simulink model "quadplane_control_dev"  (R2023a)
settings: Solver=FixedStepAuto  StartTime=0.0  StopTime=10.0  FixedStep=0.01  RelTol=1e-3
undefined symbols (not defined in the file or in its folder): Aircraft, DiscIntNeverNeededParam, framePeriod_s, frameRate_hz, InitCond
libraries: simulink x8, eeGeneralControl x6, slpidlib x3, fuzblock x1
(part 3 of 3)

== matlab function quadplane_control_dev/LowPass Filter2/LP Filter on throttle outputs/MATLAB Function ==
  data: prev_val input single; raw_val input; filtered_val output; freq_cut input; samp_freq input
function filtered_val = IIR_filt( prev_val,raw_val, freq_cut, samp_freq)
    fc = freq_cut/samp_freq;
    b = 2 - cos(2 * pi * fc) - sqrt((2 - cos(2 * pi * fc))^2 - 1);
    a = 1 - b;
    filtered_val = a * raw_val + b * prev_val;

== matlab function quadplane_control_dev/Hover Inner Loop/INDI inner loop/MATLAB Function ==
  data: B0_mat input; motor_cmds output; x_ref_rate input; Kp_term input; x_rate input
function motor_cmds = indi_inner_control(B0_mat, x_ref_rate, Kp_term, x_rate)

% INDI output change equation
motor_cmds = B0_mat \ (-x_rate + Kp_term + x_ref_rate);

== matlab function quadplane_control_dev/Hover Inner Loop/INDI inner loop/MATLAB Function1 ==
  data: mass input; cg_pos input; thrust_coefs input; B0_mat output; torque_coefs input; motor_pos input; new_inertia_inv input; motor_cmds input
function B0_mat = inversion_matrix(mass, cg_pos, thrust_coefs, torque_coefs, motor_pos, new_inertia_inv, motor_cmds)
% Included all moments modelled for hover flight

% Assumed thrust coefficient and torque coefficients are 2nd order. 
moment_arm = motor_pos - cg_pos';

% 2*a1*omega_i + a2
dummy_term = 2 * thrust_coefs(1) .* motor_cmds' + thrust_coefs(2);

% dummy term with respective y position of motor
row_1_term = - moment_arm(1:4, 2)' .* dummy_term;

% dummy term with respective x position of motor
row_2_term = moment_arm(1:4, 1)' .* dummy_term;

% 2*b1*omega_i + b2
row_3_term = [-1,-1,1,1] .* (2 * torque_coefs(1) .* motor_cmds' + torque_coefs(2));

% (-1/m)(2a1*omega_i+a2)
row_4_term = (-1/mass) * (dummy_term);

% inversion matrix for INDI
B0_mat = new_inertia_inv * [row_1_term; row_2_term; row_3_term; row_4_term];

== matlab function quadplane_control_dev/Frame Conversion ==
  data: ned_vector input; rpy_euler input; body_vector output
function body_vector = ned2body(ned_vector, rpy_euler)

roll = rpy_euler(1);
pitch = rpy_euler(2);
yaw = rpy_euler(3);

% Rotation matrix from NED to Body frame
C_ned2body = [cos(pitch)*cos(yaw), cos(pitch)*sin(yaw), -sin(pitch); ...
    sin(roll)*sin(pitch)*cos(yaw)-cos(roll)*sin(yaw), ...
    sin(roll)*sin(pitch)*sin(yaw)+cos(roll)*cos(yaw), sin(roll)*cos(pitch);...
    cos(roll)*sin(pitch)*cos(yaw)+sin(roll)*sin(yaw), ...
    cos(roll)*sin(pitch)*sin(yaw)-sin(roll)*cos(yaw), cos(roll)*cos(pitch)];

body_vector = C_ned2body * ned_vector;
